simulink model "qss_hybrid_electric_vehicle_template_1"  (R2024b)
settings: Solver=VariableStepDiscrete  StartTime=0.0  StopTime=1220  RelTol=1e-3  EnableMultiTasking=on
undefined symbols (not defined in the file): eta_EM_map, h, H_u, PMGB_NEDC, rho_f, T_CE_max, T_EM_max, V_CE_map, w_CE_max, w_EM_row
libraries: qss_tb_library x7, mpclib x1, dspindex x1
settings Model: Creator=d_goerges  LastModifiedBy=mohammed omrez khan
settings SolverCC: AlgebraicLoopSolver=TrustRegion
settings DataIOCC: LimitDataPoints=on  SaveFormat=Array  SignalLoggingSaveFormat=ModelDataLogs  ReturnWorkspaceOutputs=off
settings OptimizationCC: ExpressionDepthLimit=2147483647  LifeSpan=inf
settings DebuggingCC: UnderspecifiedInitializationDetection=Classic  MergeDetectMultiDrivingBlocksExec=none  SolverPrmCheckMsg=warning  FcnCallInpInsideContextMsg=warning  UnconnectedInputMsg=warning  UnconnectedOutputMsg=warning  UnconnectedLineMsg=warning  StateNameClashWarn=warning  SFUnexpectedBacktrackingDiag=warning  SFNoUnconditionalDefaultTransitionDiag=warning  SFExecutionAtInitializationDiag=none  ArithmeticOperatorsInVariantConditions=warning
settings HardwareCC: ProdBitPerPointer=32  ProdBitPerSizeT=32  ProdBitPerPtrDiffT=32  ProdLargestAtomicFloat=None  ProdIntDivRoundTo=Undefined  ProdEndianess=Unspecified  ProdWordSize=32  ProdHWDeviceType=32-bit Generic
settings ModelReferenceCC: PropagateSignalLabelsOutOfModel=off
settings SFSimCC: SimUseLocalCustomCode=off  CustomCodeUndefinedFunction=UseInterfaceOnly
settings RTWCC: RTWUseLocalCustomCode=off  GPUComputeCapability=3.5
settings CodeAppCC: StateflowObjectComments=on
settings GRTTargetCC: TargetLangStandard=C89/C90 (ANSI)  CombineOutputUpdateFcns=off  GRTInterface=on
settings ConfigComp: CovMetricSettings=dw  CovSaveCumulativeToWorkspaceVar=on  CovSaveSingleToWorkspaceVar=on  CovExternalEMLEnable=off

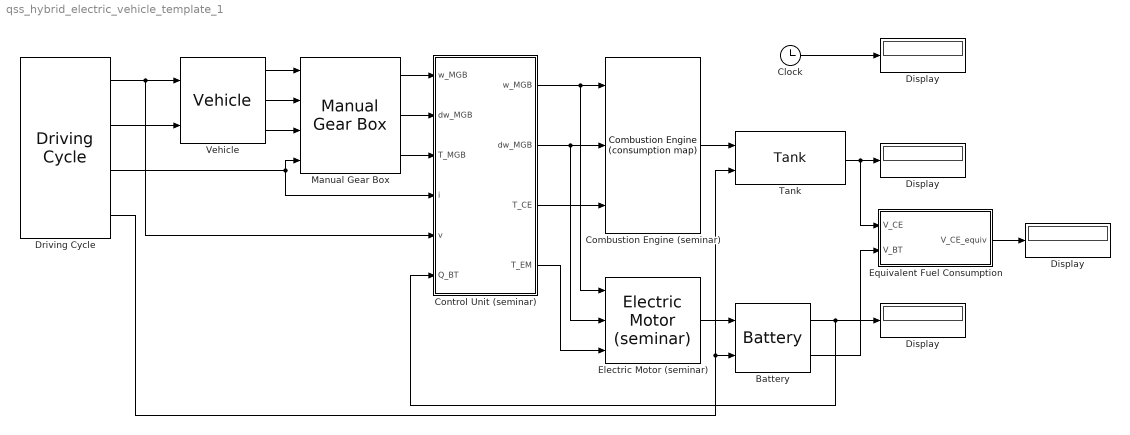
== system qss_hybrid_electric_vehicle_template_1 ==
  "   Display   " : Display
  "  Display  " : Display
  " Display " : Display
  Battery : qss_tb_library/Energy Buffer/Battery  Tag=battery  I_0=10  Q_BT_IC_rel=50  t_ch=2
  Clock : Clock
  Combustion Engine (seminar) : qss_tb_library/Energy Converter/Combustion Engine (consumption map)  Tag=combustion engine  theta_CE=0.2  w_CE_idle=105  P_CE_idle=8000  P_aux=0  ENABLE_FUEL_CUTOFF=on  T_CE_cutoff=5  P_CE_cutoff=0
  Control Unit (seminar) : Subsystem  Tag=control unit  mask(Control Unit){}
      mask help:
      | This block gives the user the opportunity to design his/her own control unit.
      |
      | The user can define the inputs and outputs  by himself/herself.
      mask init:
      | %init_control_unit;
  Display : Display
  Driving Cycle : qss_tb_library/Driving Cycle/Driving Cycle  Tag=cycle  cyclenr=Europe: NEDC  stepsize=1  autostop=on
  Electric Motor (seminar) : qss_tb_library/Energy Converter/Electric Motor (seminar)  theta_EM=0.1  P_aux=0
  Equivalent Fuel Consumption : Subsystem  mask(Equivalent Fuel Consumption){eta_BT=0.9, eta_EM=0.8, eta_CE=0.25}
      mask prompts: eta_BT "Battery efficiency [-]"; eta_EM "Motor efficiency [-]"; eta_CE "Engine efficiency [-]"
      mask help:
      | This block computes the equivalent fuel consumption.
      |
      | Input:
      | =====
      | 	V_CE    Fuel consumption [l/100 km]
      | 	V_BT    Energy consumption [kWh/100 km]
      |
      | Output:
      | ======
      | 	V_CE_equiv	Equivalent fuel consumption [l/100 km]
      mask init:
      | init_equivalent_fuel_consumption;
  Manual Gear Box : qss_tb_library/Gear System/Manual Gear Box  Tag=transmission  i_1=3.27  i_2=1.92  i_3=1.26  i_4=0.88  i_5=0.7  i_diff=3.29  e_GT=0.98  P_GT0=100  w_wheel_min=1
  Tank : qss_tb_library/Energy Source/Tank  Tag=tank  fuel=Diesel  flag_cold_start=on
  Vehicle : qss_tb_library/Vehicle/Vehicle  Tag=vehicle  m_f=1115  mt2m_f=5  A_f=2.3  d_wheel=0.576  cw=0.31  mu=0.013
  wires:
  Tank/1 -> Display/1, Equivalent Fuel Consumption/1(V_CE)
  Driving Cycle/2 -> Vehicle/2
  Driving Cycle/1 -> Vehicle/1, Control Unit (seminar)/5(v)
  Vehicle/1 -> Manual Gear Box/1
  Vehicle/2 -> Manual Gear Box/2
  Vehicle/3 -> Manual Gear Box/3
  Manual Gear Box/1 -> Control Unit (seminar)/1(w_MGB)
  Manual Gear Box/2 -> Control Unit (seminar)/2(dw_MGB)
  Manual Gear Box/3 -> Control Unit (seminar)/3(T_MGB)
  Control Unit (seminar)/1(" w_MGB ") -> Combustion Engine (seminar)/1, Electric Motor (seminar)/1
  Control Unit (seminar)/2(" dw_MGB ") -> Combustion Engine (seminar)/2, Electric Motor (seminar)/2
  Control Unit (seminar)/3(T_CE) -> Combustion Engine (seminar)/3
  Control Unit (seminar)/4(T_EM) -> Electric Motor (seminar)/3
  Combustion Engine (seminar)/1 -> Tank/1
  Electric Motor (seminar)/1 -> Battery/1
  Driving Cycle/4 -> Battery/2, Tank/2
  Battery/1 -> "  Display  "/1, Control Unit (seminar)/6(Q_BT)
  Driving Cycle/3 -> Manual Gear Box/4, Control Unit (seminar)/4(i)
  Battery/2 -> Equivalent Fuel Consumption/2(V_BT)
  Clock/1 -> " Display "/1
  Equivalent Fuel Consumption/1(V_CE_equiv) -> "   Display   "/1

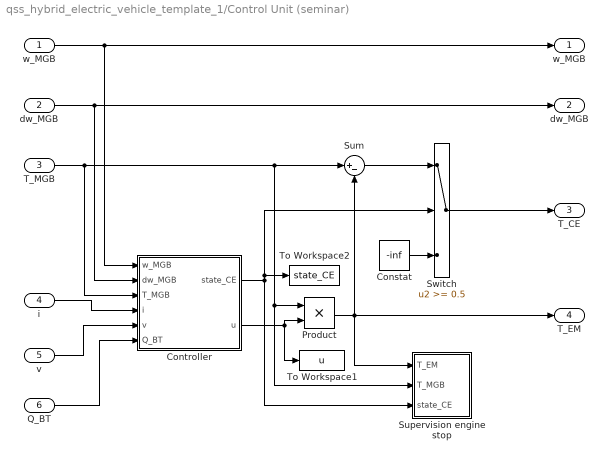
== system qss_hybrid_electric_vehicle_template_1/Control Unit (seminar) ==
  w_MGB : Inport
  dw_MGB : Inport  Port=2
  T_MGB : Inport  Port=3
  i : Inport  Port=4
  v : Inport  Port=5
  Q_BT : Inport  Port=6
  Constat : Constant  Value=-inf
  Controller : Subsystem  TreatAsAtomicUnit=on
  Product : Product  RndMeth=Zero
  Sum : Sum  Inputs=|+-
  Supervision engine stop : Subsystem
  Switch : Switch  Threshold=0.5  SaturateOnIntegerOverflow=off  InputSameDT=off
  To Workspace1 : ToWorkspace  VariableName=u  SampleTime=-1
  To Workspace2 : ToWorkspace  VariableName=state_CE  SampleTime=-1
  " w_MGB " : Outport  InitialOutput=0
  " dw_MGB " : Outport  Port=2  InitialOutput=0
  T_CE : Outport  Port=3  InitialOutput=0
  T_EM : Outport  Port=4  InitialOutput=0
  wires:
  dw_MGB/1 -> Controller/2(dw_MGB), " dw_MGB "/1
  w_MGB/1 -> Controller/1(w_MGB), " w_MGB "/1
  T_MGB/1 -> Controller/3(T_MGB), Sum/1, Product/1, Supervision engine stop/2(T_MGB)
  Product/1 -> Sum/2, T_EM/1, Supervision engine stop/1(T_EM)
  Controller/2(u) -> Product/2, To Workspace1/1
  i/1 -> Controller/4(i)
  Controller/1(state_CE) -> Switch/2, To Workspace2/1, Supervision engine stop/3(state_CE)
  Sum/1 -> Switch/1
  Switch/1 -> T_CE/1
  Constat/1 -> Switch/3
  v/1 -> Controller/5(v)
  Q_BT/1 -> Controller/6(Q_BT)

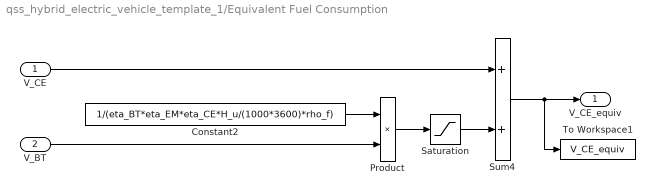
== system qss_hybrid_electric_vehicle_template_1/Equivalent Fuel Consumption ==
  V_CE : Inport
  V_BT : Inport  Port=2
  Constant2 : Constant  Value=1/(eta_BT*eta_EM*eta_CE*H_u/(1000*3600)*rho_f)
  Product : Product  RndMeth=Zero
  Saturation : Saturate  UpperLimit=inf  LowerLimit=0
  Sum4 : Sum  InputSameDT=on  SaturateOnIntegerOverflow=on  OutDataTypeStr=Inherit: Same as first input
  To Workspace1 : ToWorkspace  VariableName=V_CE_equiv  SampleTime=-1
  V_CE_equiv : Outport
  wires:
  Product/1 -> Saturation/1
  V_BT/1 -> Product/2
  Constant2/1 -> Product/1
  Sum4/1 -> To Workspace1/1, V_CE_equiv/1
  V_CE/1 -> Sum4/1
  Saturation/1 -> Sum4/2

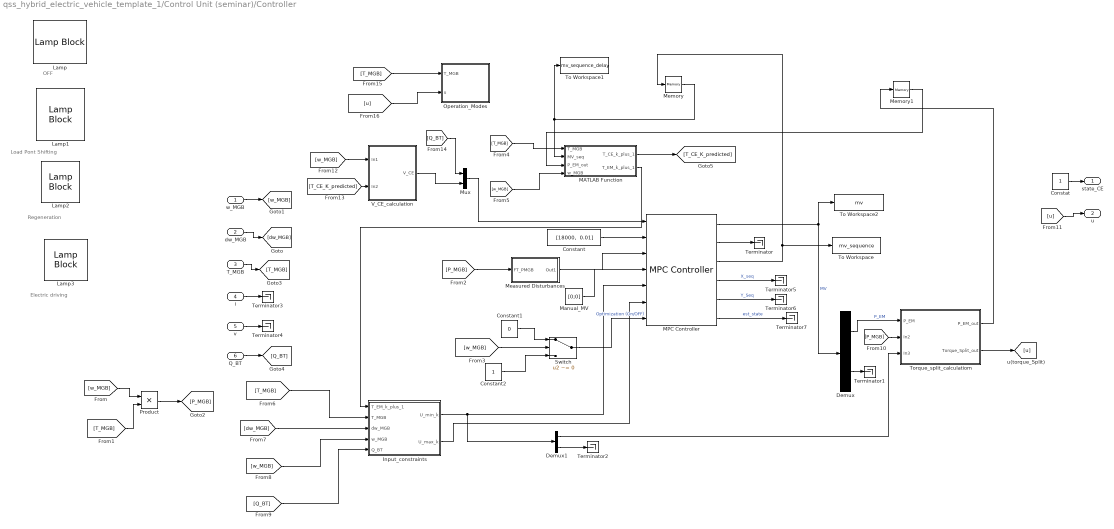
== system qss_hybrid_electric_vehicle_template_1/Control Unit (seminar)/Controller ==
  note: OFF
  note: Load Pont Shifting
  note: Regeneration
  note: Electric driving
  w_MGB : Inport
  dw_MGB : Inport  Port=2
  T_MGB : Inport  Port=3
  i : Inport  Port=4
  v : Inport  Port=5
  Q_BT : Inport  Port=6
  Constant : Constant  Value="[18000,  0.01]"
  Constant1 : Constant  Value=0
  Constant2 : Constant
  Constat : Constant
  Demux : Demux  Outputs=2
  Demux1 : Demux  Outputs=2
  Input_constraints : Subsystem
  Lamp{,1..3} (4 alike) : LampBlock  LabelPosition=Hide
  MATLAB Function : MATLAB Function  TreatAsAtomicUnit=on
  MPC Controller : mpclib/MPC Controller  SCDEnableBlockLinearizationSpecification=on  mpcobj=mpc_object  is_multiple=0  enable_value=0  return_u0=off  updateMPCinCallerWorkspace=on  md_inport=on  mv_inport=on  uref_inport=off  return_cost=on  return_mvseq=on  return_qpstatus=off  return_xseq=on  return_state=on  return_ovseq=on  state_inport=off  umin_inport=on  umax_inport=on  ymin_inport=off  ymax_inport=off  cc_inport=off  ywt_inport=off  uwt_inport=off  duwt_inport=off  rhoeps_inport=off  pm_inport=off  MaximumP=10  HorizonChoice=FixedHorizon  n_ts=1  n_p=11  n_mv=2  n_md=1  n_ud=0  n_mo=2  n_uo=0  BlockDataType=double  SampleTimeInherited=off  switch_inport=on
  Manual_MV : Constant  Value=[0;0]  VectorParams1D=off
  "Measured Disturbances " : Subsystem
  Memory : Memory
  Memory1 : Memory
  Mux : Mux  Inputs=2
  Operation_Modes : Stateflow chart  TreatAsAtomicUnit=on
  Product : Product
  Switch : Switch  Criteria=u2 ~= 0  SaturateOnIntegerOverflow=off  InputSameDT=off
  Terminator{,1..7} (8 alike) : Terminator
  To Workspace : ToWorkspace  VariableName=mv_sequence  SaveFormat=Timeseries  SampleTime=-1
  To Workspace1 : ToWorkspace  VariableName=mv_sequence_delay  SaveFormat=Timeseries  SampleTime=-1
  To Workspace2 : ToWorkspace  VariableName=mv  SaveFormat=Timeseries  SampleTime=-1
  Torque_split_calculatiom : Subsystem
  V_CE_calculation : Subsystem
  state_CE : Outport  InitialOutput=0
  u : Outport  Port=2  InitialOutput=0
  wires:
  w_MGB/1 -> [w_MGB]
  dw_MGB/1 -> [dw_MGB]
  T_MGB/1 -> [T_MGB]
  i/1 -> Terminator3/1
  [u] -> u/1
  Constat/1 -> state_CE/1
  v/1 -> Terminator4/1
  Q_BT/1 -> [Q_BT]
  [w_MGB] -> Product/1
  [T_MGB] -> Product/2
  Product/1 -> [P_MGB]
  [P_MGB] -> "Measured Disturbances "/1(FT_PMGB)
  "Measured Disturbances "/1(Out1) -> MPC Controller/3
  Constant/1 -> MPC Controller/2
  Manual_MV/1 -> MPC Controller/4
  [w_MGB] -> Switch/2
  Constant1/1 -> Switch/1
  Constant2/1 -> Switch/3
  Switch/1 -> MPC Controller/7  "Optimization (On/OFF)"
  [T_MGB] -> MATLAB Function/1(T_MGB)
  [w_MGB] -> MATLAB Function/4(w_MGB)
  MATLAB Function/1(T_CE_k_plus_1) -> [T_CE_K_predicted]
  MPC Controller/2 -> Terminator/1
  MPC Controller/3 -> To Workspace/1, Memory/1
  Memory/1 -> MATLAB Function/2(MV_seq), To Workspace1/1
  MATLAB Function/2(T_EM_k_plus_1) -> Input_constraints/1(T_EM_k_plus_1)
  [T_MGB] -> Input_constraints/2(T_MGB)
  [dw_MGB] -> Input_constraints/3(dw_MGB)
  [w_MGB] -> Input_constraints/4(w_MGB)
  [Q_BT] -> Input_constraints/5(Q_BT)
  Input_constraints/1(U_min_k) -> Demux1/1, MPC Controller/5
  Input_constraints/2(U_max_k) -> MPC Controller/6
  MPC Controller/1 -> To Workspace2/1, Demux/1  "MV"
  Demux1/2 -> Terminator2/1
  Memory1/1 -> MATLAB Function/3(P_EM_out)
  Demux/1 -> Torque_split_calculatiom/1(P_EM)  "P_EM"
  [P_MGB] -> Torque_split_calculatiom/2(In2)
  Demux1/1 -> Torque_split_calculatiom/3(In3)
  Torque_split_calculatiom/1(P_EM_out) -> Memory1/1
  Torque_split_calculatiom/2(Torque_Split_out) -> [u]
  MPC Controller/4 -> Terminator5/1  "X_seq"
  MPC Controller/5 -> Terminator6/1  "Y_Seq"
  MPC Controller/6 -> Terminator7/1  "est_state"
  Demux/2 -> Terminator1/1
  [Q_BT] -> Mux/1
  [w_MGB] -> V_CE_calculation/1(In1)
  [T_CE_K_predicted] -> V_CE_calculation/2(In2)
  V_CE_calculation/1(V_CE) -> Mux/2
  Mux/1 -> MPC Controller/1
  [u] -> Operation_Modes/2(u)
  [T_MGB] -> Operation_Modes/1(T_MGB)

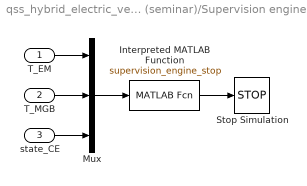
== system qss_hybrid_electric_vehicle_template_1/Control Unit (seminar)/Supervision engine stop ==
  T_EM : Inport
  T_MGB : Inport  Port=2
  state_CE : Inport  Port=3
  Interpreted MATLAB Function : MATLABFcn  MATLABFcn=supervision_engine_stop
  Mux : Mux  Inputs=3
  Stop Simulation : Stop
  wires:
  T_MGB/1 -> Mux/2
  T_EM/1 -> Mux/1
  state_CE/1 -> Mux/3
  Mux/1 -> Interpreted MATLAB Function/1
  Interpreted MATLAB Function/1 -> Stop Simulation/1

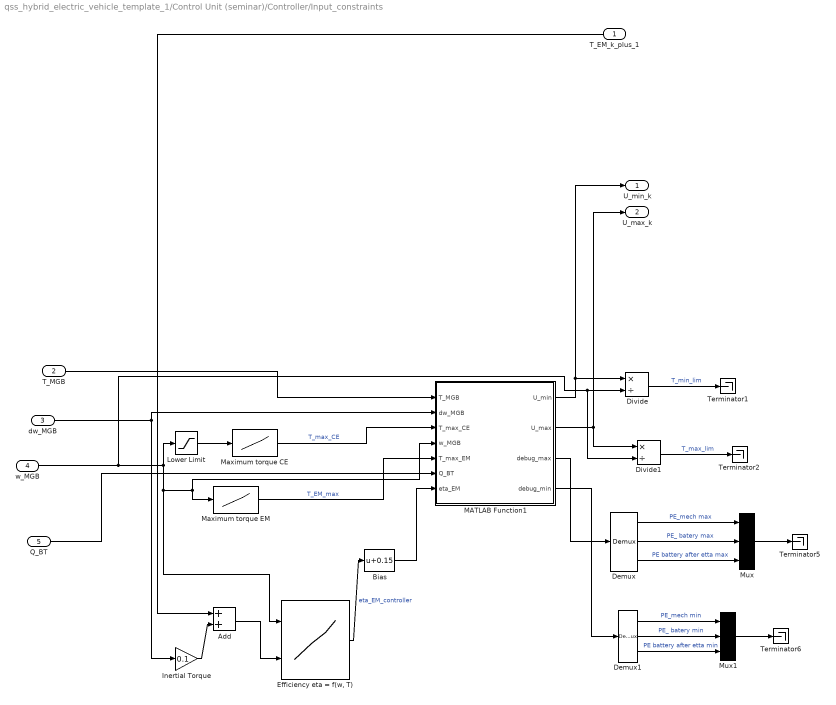
== system qss_hybrid_electric_vehicle_template_1/Control Unit (seminar)/Controller/Input_constraints ==
  T_EM_k_plus_1 : Inport
  T_MGB : Inport  Port=2
  dw_MGB : Inport  Port=3
  w_MGB : Inport  Port=4
  Q_BT : Inport  Port=5
  Add : Sum
  Bias : Bias  Bias=0.15  SaturateOnIntegerOverflow=off
  Demux : Demux  Outputs=3
  Demux1 : Demux  Outputs=3
  Divide : Product  Inputs=*/
  Divide1 : Product  Inputs=*/
  "Efficiency eta = f(w, T)" : Lookup2D  RowIndex=w_EM_row  ColumnIndex=T_EM_col  Table=eta_EM_map  InputSameDT=off
  Inertial Torque : Gain  Gain=0.1
  Lower Limit : Saturate  UpperLimit=inf  LowerLimit=105
  MATLAB Function1 : MATLAB Function  TreatAsAtomicUnit=on
  Maximum torque CE : Lookup  InputValues=w_CE_max  Table=T_CE_max
  Maximum torque EM : Lookup  InputValues=w_EM_row  Table=T_EM_max
  Mux : Mux  Inputs=3
  Mux1 : Mux  Inputs=3
  Terminator{1..2,5..6} (4 alike) : Terminator
  U_min_k : Outport
  U_max_k : Outport  Port=2
  wires:
  "Efficiency eta = f(w, T)"/1 -> Bias/1  "eta_EM_controller"
  w_MGB/1 -> Divide1/2, Divide/2, "Efficiency eta = f(w, T)"/1, Maximum torque EM/1, MATLAB Function1/4(w_MGB), Lower Limit/1
  Q_BT/1 -> MATLAB Function1/6(Q_BT)
  Inertial Torque/1 -> Add/2
  Add/1 -> "Efficiency eta = f(w, T)"/2
  Maximum torque EM/1 -> MATLAB Function1/5(T_max_EM)  "T_EM_max"
  Divide/1 -> Terminator1/1  "T_min_lim"
  MATLAB Function1/1(U_min) -> U_min_k/1, Divide/1
  Divide1/1 -> Terminator2/1  "T_max_lim"
  Maximum torque CE/1 -> MATLAB Function1/3(T_max_CE)  "T_max_CE"
  Lower Limit/1 -> Maximum torque CE/1
  Demux/2 -> Mux/2  "PE_ batery max"
  MATLAB Function1/2(U_max) -> U_max_k/1, Divide1/1
  dw_MGB/1 -> Inertial Torque/1, MATLAB Function1/2(dw_MGB)
  Bias/1 -> MATLAB Function1/7(eta_EM)
  Demux/3 -> Mux/3  "PE battery after etta max"
  MATLAB Function1/3(debug_max) -> Demux/1
  Mux/1 -> Terminator5/1
  MATLAB Function1/4(debug_min) -> Demux1/1
  Mux1/1 -> Terminator6/1
  Demux1/1 -> Mux1/1  "PE_mech min"
  Demux1/2 -> Mux1/2  "PE_ batery min"
  Demux1/3 -> Mux1/3  "PE battery after etta min"
  Demux/1 -> Mux/1  "PE_mech max"
  T_MGB/1 -> MATLAB Function1/1(T_MGB)
  T_EM_k_plus_1/1 -> Add/1

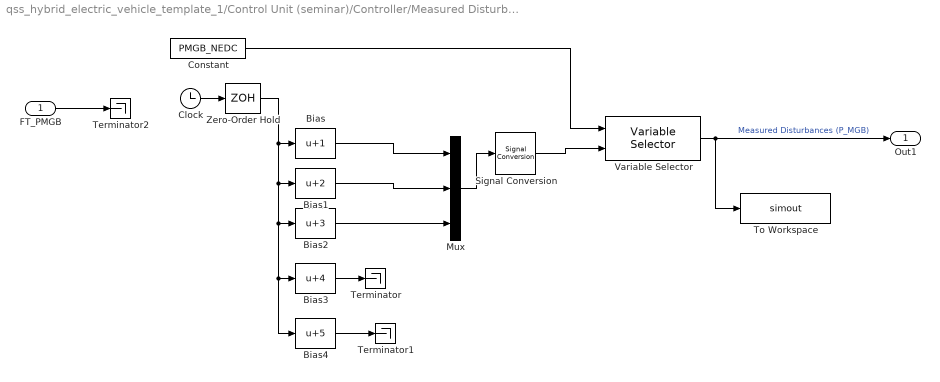
== system qss_hybrid_electric_vehicle_template_1/Control Unit (seminar)/Controller/Measured Disturbances  ==
  FT_PMGB : Inport
  Bias : Bias  Bias=1  SaturateOnIntegerOverflow=off
  Bias1 : Bias  Bias=2  SaturateOnIntegerOverflow=off
  Bias2 : Bias  Bias=3  SaturateOnIntegerOverflow=off
  Bias3 : Bias  Bias=4  SaturateOnIntegerOverflow=off
  Bias4 : Bias  Bias=5  SaturateOnIntegerOverflow=off
  Clock : Clock
  Constant : Constant  Value=PMGB_NEDC
  Mux : Mux  Inputs=3
  Signal Conversion : SignalConversion  OverrideOpt=off
  Terminator : Terminator
  Terminator1 : Terminator
  Terminator2 : Terminator
  To Workspace : ToWorkspace  VariableName=simout  SaveFormat=Timeseries  SampleTime=-1
  Variable Selector : dspindex/Variable Selector  NumInputs=1  rowsOrCols=Rows  IdxMode=Variable  Elements=[1 3]  ZerOneIdxMode=One-based  errmode=Clip Index  FillMode=on  FillValues=0
  Zero-Order Hold : ZeroOrderHold  SampleTime=-1
  Out1 : Outport
  wires:
  Constant/1 -> Variable Selector/1
  Bias2/1 -> Mux/3
  Bias3/1 -> Terminator/1
  Zero-Order Hold/1 -> Bias4/1, Bias3/1, Bias2/1, Bias1/1, Bias/1
  FT_PMGB/1 -> Terminator2/1
  Bias4/1 -> Terminator1/1
  Signal Conversion/1 -> Variable Selector/2
  Bias/1 -> Mux/1
  Mux/1 -> Signal Conversion/1
  Bias1/1 -> Mux/2
  Clock/1 -> Zero-Order Hold/1
  Variable Selector/1 -> To Workspace/1, Out1/1  "Measured Disturbances (P_MGB)"

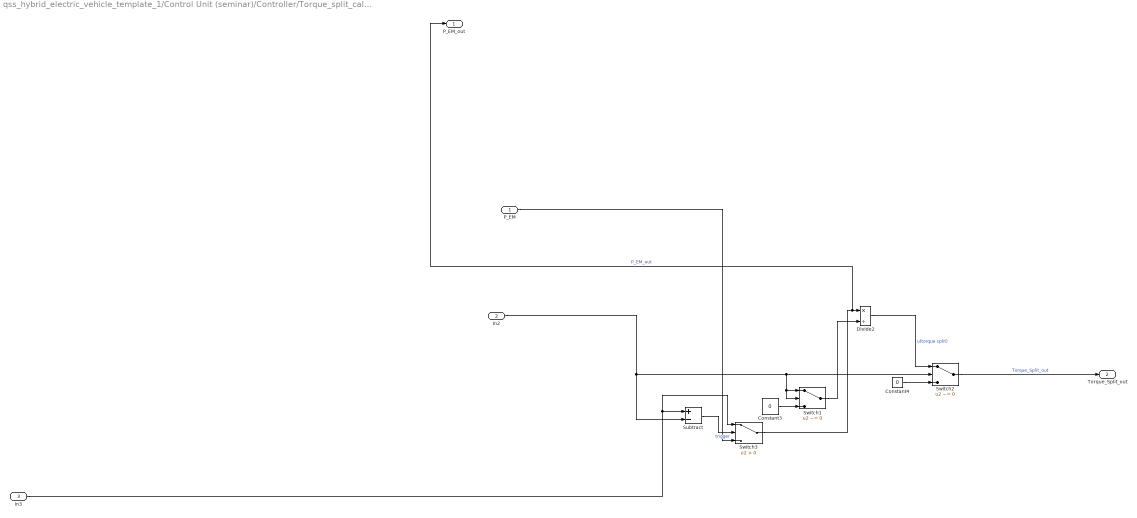
== system qss_hybrid_electric_vehicle_template_1/Control Unit (seminar)/Controller/Torque_split_calculatiom ==
  P_EM : Inport
  In2 : Inport  Port=2
  In3 : Inport  Port=3
  Constant3 : Constant  Value=0
  Constant4 : Constant  Value=0
  Divide2 : Product  Inputs=*/
  Subtract : Sum  Inputs=+-
  Switch1 : Switch  Criteria=u2 ~= 0  SaturateOnIntegerOverflow=off  InputSameDT=off
  Switch2 : Switch  Criteria=u2 ~= 0  SaturateOnIntegerOverflow=off  InputSameDT=off
  Switch3 : Switch  Criteria=u2 > Threshold  SaturateOnIntegerOverflow=off  InputSameDT=off
  P_EM_out : Outport
  Torque_Split_out : Outport  Port=2
  wires:
  In2/1 -> Subtract/2, Switch1/2, Switch1/1, Switch2/2
  In3/1 -> Switch3/1, Subtract/1
  Divide2/1 -> Switch2/1  "u(torque split)"
  Switch3/1 -> P_EM_out/1, Divide2/1  "P_EM_out"
  Switch1/1 -> Divide2/2
  Constant3/1 -> Switch1/3
  Constant4/1 -> Switch2/3
  Subtract/1 -> Switch3/2  "trigger"
  P_EM/1 -> Switch3/3
  Switch2/1 -> Torque_Split_out/1  "Torque_Split_out"

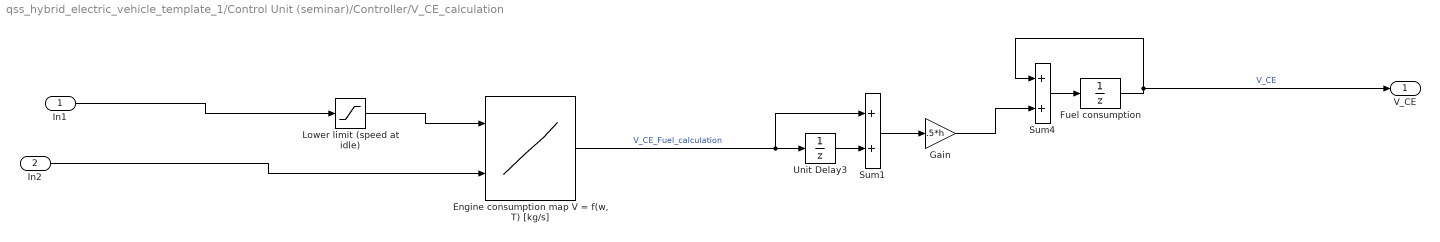
== system qss_hybrid_electric_vehicle_template_1/Control Unit (seminar)/Controller/V_CE_calculation ==
  In1 : Inport
  In2 : Inport  Port=2
  "Engine consumption map V = f(w, T) [kg/s]" : Lookup2D  RowIndex=w_CE_row  ColumnIndex=T_CE_col  Table=V_CE_map  SaturateOnIntegerOverflow=off  InputSameDT=off
  Fuel consumption : UnitDelay  SampleTime=h  HasFrameUpgradeWarning=on
  Gain : Gain  Gain=.5*h
  Lower limit (speed at idle) : Saturate  UpperLimit=inf  LowerLimit=105
  Sum1 : Sum  InputSameDT=on  SaturateOnIntegerOverflow=on  OutDataTypeStr=Inherit: Same as first input
  Sum4 : Sum  InputSameDT=on  SaturateOnIntegerOverflow=on  OutDataTypeStr=Inherit: Same as first input
  Unit Delay3 : UnitDelay  SampleTime=h  HasFrameUpgradeWarning=on
  V_CE : Outport
  wires:
  Sum1/1 -> Gain/1
  "Engine consumption map V = f(w, T) [kg/s]"/1 -> Sum1/1, Unit Delay3/1  "V_CE_Fuel_calculation"
  Fuel consumption/1 -> V_CE/1, Sum4/1  "V_CE"
  Unit Delay3/1 -> Sum1/2
  Sum4/1 -> Fuel consumption/1
  Lower limit (speed at idle)/1 -> "Engine consumption map V = f(w, T) [kg/s]"/1
  Gain/1 -> Sum4/2
  In2/1 -> "Engine consumption map V = f(w, T) [kg/s]"/2
  In1/1 -> Lower limit (speed at idle)/1

== matlab function qss_hybrid_electric_vehicle_template_1/Control Unit (seminar)/Controller/Input_constraints/MATLAB Function1 ==
  data: T_MGB input; U_min output; dw_MGB input; T_max_CE input; w_MGB input; T_max_EM input; Q_BT input; eta_EM input; U_max output; debug_max output; debug_min output
function [U_min,U_max,debug_max,debug_min] = Input_Constraints(T_MGB, dw_MGB, T_max_CE, w_MGB, T_max_EM, Q_BT, eta_EM)


delta_t = 1;
delta_p = delta_t * w_MGB;
theta_CE = 0.2;
theta_EM = 0.1;


% Battery Parameters
c_BT_E1     =  39;                          % Minimum battery voltage for discharging (13 cells, 3 V/cell, seminar)                 [V]
c_BT_E2     =  0.013;					    % Minimum battery resistance for discharging (13 cells, 1 mOhm/cell, seminar)           [Ohm]
c_BT_E3     =  15.6;					    % Maximum battery voltage variation for discharging (13 cells, 1.2 V/cell, seminar)     [V]
c_BT_E4     =  0;							% Minimum battery resistance variation for discharging (13 cells, 0 mOhm/cell, seminar) [Ohm]
c_BT_L1     =  c_BT_E1;                     % c_BT_L1 = c_BT_EL1 for continuity reasons
c_BT_L2     =  0.013;					    % Minimum battery resistance for charging (13 cells, 1 mOhm/cell, seminar)              [V]
c_BT_L3     =  c_BT_E3;                     % c_BT_L3 = c_BT_EL3 for continuity reasons
c_BT_L4     =  0.00;                        % Minimum battery resistance variation for charging (13 cells, 0 mOhm/cell, seminar)    [Ohm]

I_0 = 10;

Q_bt0      = I_0 * 3600;					% Discharge current in 1 h              [C]
I_bt_max    = (60/2)*I_0;			    	% Maximum charge/discharge current      [A]
%eta_EM = 1; 

%%
% During discharging 
AE1_discharge = (c_BT_E3 * (Q_BT/Q_bt0)) + c_BT_E1;
AE2_discharge = (c_BT_E4) * (Q_BT/Q_bt0) + c_BT_E2;
P_BT_discharge = I_bt_max^2 * ((AE1_discharge/I_bt_max) - (AE2_discharge/I_0));

% During charging
AE1_charge = (c_BT_L3 * (Q_BT/Q_bt0)) + c_BT_L1;
AE2_charge = (c_BT_L4) * (Q_BT/Q_bt0) + c_BT_L2;
P_BT_charge = -(I_bt_max^2 * ((AE1_charge/I_bt_max) - (AE2_charge/I_0)));




%% CE Constraints
T_CE_inertia = abs(theta_CE* dw_MGB);       % Inertial Torque of CE
% Upper Limit of P_CE
T_CE_upper = T_max_CE-delta_t -T_CE_inertia;
P_CE_max = T_CE_upper*w_MGB;

% Lower Limit of P_CE 
P_CE_min = 0;
  

%% EM Constraints

T_EM_inertia = abs(theta_EM* dw_MGB);
% Upper Limit of P_EM

    if w_MGB > 0
        T_EM_upper = T_max_EM - T_EM_inertia - delta_t;
    else
        T_EM_upper = T_max_EM -T_EM_inertia;                % delta is not include because at w_MGB =0, T_EM should be 0
    end
    
P_EM_lim_max = T_EM_upper * w_MGB;
P_em_cur_max = P_BT_discharge/eta_EM - (T_EM_inertia * w_MGB);
P_EM_max = min(P_EM_lim_max,P_em_cur_max-delta_p);


% Lower Limit of P_EM
if T_MGB >=0
    T_EM_lower = -T_EM_upper;
else
    T_EM_lower = max(T_MGB+delta_t, -T_EM_upper);
end

P_EM_lim_min = T_EM_lower * w_MGB;


P_em_cur_min = P_BT_charge/eta_EM -(T_EM_inertia*w_MGB);
P_EM_min = max(P_EM_lim_min,P_em_cur_min+delta_p);

debug_max = [P_EM_lim_max,P_BT_discharge,P_em_cur_max];
debug_min = [P_EM_lim_min,P_BT_charge,P_em_cur_min];
U_min = [P_EM_min;P_CE_min];
U_max = [P_EM_max;P_CE_max];

== matlab function qss_hybrid_electric_vehicle_template_1/Control Unit (seminar)/Controller/MATLAB Function ==
  data: T_MGB input; T_CE_k_plus_1 output; MV_seq input; P_EM_out input; w_MGB input; T_EM_k_plus_1 output
function [T_CE_k_plus_1,T_EM_k_plus_1] = fcn(T_MGB, MV_seq,P_EM_out, w_MGB)
T_EM_k_plus_1 = 0;
PCE_K_plus_1 = MV_seq(2,2);
PEM_K_plus_1 = MV_seq(2,1);
if w_MGB > 105
    T_CE_k_plus_1 = PCE_K_plus_1/w_MGB;
else
    T_CE_k_plus_1 = 0;
end
if T_MGB >=0
    if w_MGB == 0
        T_EM_k_plus_1 = 0;
    else 
        T_EM_k_plus_1 = PEM_K_plus_1/w_MGB;
    end
else
    if w_MGB ~= 0
        T_EM_k_plus_1 = P_EM_out/w_MGB;
    else
    end

end

end

== stateflow chart qss_hybrid_electric_vehicle_template_1/Control Unit (seminar)/Controller/Operation_Modes ==
  state Regeneration
    entry:
    OFF_States = 0;
    LPS = 0;
    ED=0;
    REG=1;
  state Load_Point_Shifting
    entry:
    OFF_States = 0;
    LPS = 1;
    ED=0;
    REG=0;
  state OFF
    entry:
    OFF_States = 1;
    LPS = 0;
    ED=0;
    REG=0;
    OFF -> OFF [order 1]
  state Electric_Driving
    entry:
    OFF_States = 0;
    LPS = 0;
    ED=1;
    REG=0;
  Load_Point_Shifting -> Regeneration [order 2] : [(T_MGB <0 & u == 1) | (T_MGB < 0 & 0 <= u & u < 1)]
  Regeneration -> Load_Point_Shifting [order 1] : [[(T_MGB >0 & 0 <= u & u < 1) | (T_MGB > 0 & u < 0)]]
  (default) -> OFF
  Load_Point_Shifting -> OFF [order 3] : [T_MGB == 0 & u == 0]
  Regeneration -> OFF [order 3] : [T_MGB == 0 & u == 0]
  OFF -> Load_Point_Shifting [order 1] : [[(T_MGB >0 & 0 <= u & u < 1) | (T_MGB > 0 & u < 0)]]
  OFF -> Regeneration [order 2] : [[(T_MGB <0 & u == 1) | (T_MGB < 0 & 0 <= u & u < 1)]]
  Electric_Driving -> OFF [order 3] : [T_MGB == 0 & u == 0]
  OFF -> Electric_Driving [order 3] : [[T_MGB > 0 & u == 1]]
  Electric_Driving -> Load_Point_Shifting [order 2] : [(T_MGB >0 & 0 <= u & u < 1) | (T_MGB > 0 & u < 0)]
  Load_Point_Shifting -> Electric_Driving [order 1] : [T_MGB > 0 & u== 1]
  Electric_Driving -> Regeneration [order 1] : [(T_MGB <0 & u == 1) | (T_MGB < 0 & 0 <= u & u < 1)]
  Regeneration -> Electric_Driving [order 2] : [T_MGB > 0 & u == 1]
  data: T_MGB input; u input; OFF_States local; LPS local; ED local; REG local
